simulink model "EE435_project_v10"  (R2018b)
settings: Solver=VariableStepAuto  StartTime=0.0  StopTime=8/60  RelTol=1e-3
libraries: powerlib x26, simulink x4, powerlib_meascontrol x2, re_lib x1, pePowerMeasurement x1
settings Model: Creator=jmyea  LastModifiedBy=jmyea
settings SolverCC: ZeroCrossAlgorithm=Adaptive
settings DebuggingCC: MaskedZcDiagnostic=none  IgnoredZcDiagnostic=none

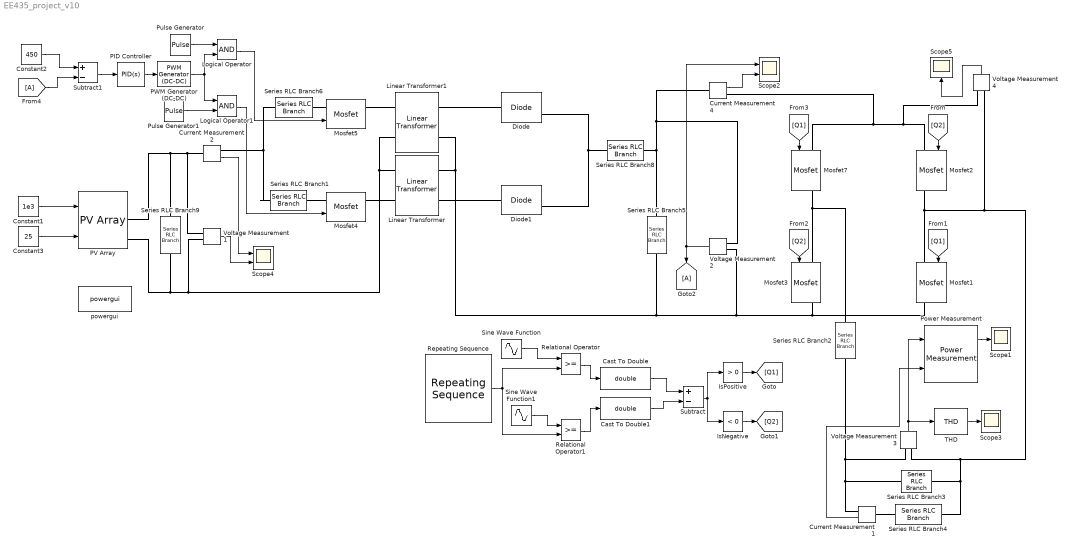
== system EE435_project_v10 ==
  Cast To Double : DataTypeConversion  OutDataTypeStr=double
  Cast To Double1 : DataTypeConversion  OutDataTypeStr=double
  Constant1 : Constant  Value=1e3
  Constant2 : Constant  Value=450
  Constant3 : Constant  Value=25
  Current Measurement1 : powerlib/Measurements/Current Measurement  PhasorSimulation=off  OutputType=Complex  PSBequivalent=0
  Current Measurement2 : powerlib/Measurements/Current Measurement  PhasorSimulation=off  OutputType=Complex  PSBequivalent=0
  Current Measurement4 : powerlib/Measurements/Current Measurement  PhasorSimulation=off  OutputType=Complex  PSBequivalent=0
  Diode : powerlib/Power Electronics/Diode  Ron=0.001  Lon=0  Vf=0.8  IC=0  UseSnubber=0  Rs=500  Cs=250e-9  Measurements=on
  Diode1 : powerlib/Power Electronics/Diode  Ron=0.001  Lon=0  Vf=0.8  IC=0  UseSnubber=0  Rs=500  Cs=250e-9  Measurements=on
  IsNegative : simulink/Logic and Bit Operations/Compare To Zero  relop=<  OutDataTypeStr=boolean
  IsPositive : simulink/Logic and Bit Operations/Compare To Zero  relop=>  OutDataTypeStr=boolean
  Linear Transformer : powerlib/Elements/Linear Transformer  UNITS=SI  NominalPower=[8.5e3 100e3]  winding1=[200 0 0]  winding2=[600 0 0]  ThreeWindings=off  winding3=[2.6e3 0 0]  RmLm=[inf inf]  Measurements=None  DataType=on
  Linear Transformer1 : powerlib/Elements/Linear Transformer  UNITS=SI  NominalPower=[8.5e3 100e3]  winding1=[200 0 0]  winding2=[600 0 0]  ThreeWindings=off  winding3=[2.6e3 0 0]  RmLm=[inf inf]  Measurements=None  DataType=on
  Logical Operator : Logic  AllPortsSameDT=off  OutDataTypeStr=boolean
  Logical Operator1 : Logic  AllPortsSameDT=off  OutDataTypeStr=boolean
  Mosfet{1..4,7} (5 alike) : powerlib/Power Electronics/Mosfet  Ron=80e-3  Lon=0  Rd=0.01  Vfd=3.5  IC=0  Rs=65.24  Cs=0.647e-6  Measurements=on
  Mosfet5 : powerlib/Power Electronics/Mosfet  Ron=80e-3  Lon=0  Rd=0.01  Vfd=3.5  IC=0  Rs=183  Cs=9.323e-9  Measurements=on
  PID Controller : simulink/Continuous/PID Controller  Controller=PID  Form=Parallel  TimeDomain=Continuous-time  SampleTime=-1  IntegratorMethod=Forward Euler  FilterMethod=Forward Euler  ControllerParametersSource=internal  P=1  I=1  D=0  UseFilter=on  N=100  TunerSelectOption=Transfer Function Based (PID Tuner App)  InitialConditionSource=internal  InitialConditionForIntegrator=0  InitialConditionForFilter=0  DifferentiatorICPrevScaledInput=0  ExternalReset=none  TrackingMode=off  Kt=1  LimitOutput=off  UpperSaturationLimit=inf  LowerSaturationLimit=-inf  LinearizeAsGain=on  AntiWindupMode=none  Kb=1  POutMin=[]  POutMax=[]  IOutMin=[]  IOutMax=[]  DOutMin=[]  DOutMax=[]  NOutMin=[]  NOutMax=[]  SumOutMin=[]  SumOutMax=[]  SaturationOutMin=[]  SaturationOutMax=[]  PParamMin=[]  PParamMax=[]  IParamMin=[]  IParamMax=[]  DParamMin=[]  DParamMax=[]  NParamMin=[]  NParamMax=[]  KbParamMin=[]  KbParamMax=[]  KtParamMin=[]  KtParamMax=[]  KbOutMin=[]  KbOutMax=[]  KtOutMin=[]  KtOutMax=[]  IntegratorOutMin=[]  IntegratorOutMax=[]  FilterOutMin=[]  FilterOutMax=[]  SumI1OutMin=[]  SumI1OutMax=[]  SumI2OutMin=[]  SumI2OutMax=[]  SumI3OutMin=[]  SumI3OutMax=[]  SumI4OutMin=[]  SumI4OutMax=[]  SumDOutMin=[]  SumDOutMax=[]  DifferentiatorOutMin=[]  DifferentiatorOutMax=[]  FilterDiffOutCoefMin=[]  FilterDiffOutCoefMax=[]  ReciprocalOutMin=[]  ReciprocalOutMax=[]  SumDenOutMin=[]  SumDenOutMax=[]  SumNumOutMin=[]  SumNumOutMax=[]  DivideOutMin=[]  DivideOutMax=[]  IntegratorContinuousStateAttributes=''  IntegratorStateMustResolveToSignalObject=off  IntegratorRTWStateStorageClass=Auto  FilterContinuousStateAttributes=''  FilterStateMustResolveToSignalObject=off  FilterRTWStateStorageClass=Auto  ParallelPVariant=InternalParameters  IdealPVariant=Disabled  IVariant=InternalParameters  DVariant=InternalParameters  IntegratorVariant=Continuous  SatVariant=Disabled  AWVariant=Passthrough  PCopyVariant=Disabled  TRVariant=Disabled  FdbkBlocksVariant=Forward  IdealPFdbkVariant=Disabled  SatFdbkVariant=Disabled  DerivativeFilterVariant=ContFilter  NVariant=InternalParameters  NCopyVariant=Disabled  FilterICVariant=InternalICsFilter  IntegratorICVariant=InternalICs  ExternalResetVariant=Disabled  TRSumVariant=Passthrough  SumFdbkVariant=Disabled  SumVariant=Sum_PID
  PV Array : re_lib/Solar/PV Array  Npar=2  Nser=5  PlotType=array @ 25 deg.C & specified irradiances  S_vec="[ 1000  500  100 ]"  Temp_C_vec="[ 45 25  ]"  ModuleName=User-defined  PlotWhenSelected=off  Pm=330.6  Ncell=60  Voc=67.7  Isc=6.07  Vm=58  Im=5.7  beta_Voc_pc=-0.276  alpha_Isc_pc=0.059  beta_Voc=-0.18685  alpha_Isc=0.0035813  IL=6.1233  I0=7.4689e-12  nI=1.6029  Rsh=328.5492  Rs=0.31806  BAL=on  Tc=1e-6  Tfilter=5e-5
  PWM Generator (DC-DC) : powerlib_meascontrol/Pulse & Signal Generators/PWM Generator (DC-DC)  Fsw=60e3  Ts=0
  Power Measurement : pePowerMeasurement/Power Measurement  LabelModeActiveChoice=Continuous  F=60  K=[0 1 2 3]  Ts=0
  Pulse Generator : DiscretePulseGenerator  PulseType=Time based  Period=1/30e3  PulseWidth=50
  Pulse Generator1 : DiscretePulseGenerator  PulseType=Time based  Period=1/30e3  PulseWidth=50  PhaseDelay=1/(2*(30e3))
  Relational Operator : RelationalOperator  OutDataTypeStr=boolean  RndMeth=Simplest
  Relational Operator1 : RelationalOperator  OutDataTypeStr=boolean  RndMeth=Simplest
  Repeating Sequence : simulink/Sources/Repeating Sequence  rep_seq_t=[0 1/(60e3) 2/(60e3) 3/(60e3) 4/(60e3)]  rep_seq_y=[1 0 -1 0 1]
  Scope1 : Scope
  Scope2 : Scope  NumInputPorts=2
  Scope3 : Scope
  Scope4 : Scope  NumInputPorts=2
  Scope5 : Scope
  Series RLC Branch1 : powerlib/Elements/Series RLC Branch  LConnTagsString=__new0  RConnTagsString=__new0  BranchType=RL  Resistance=20  Inductance=1e-3  SetiL0=off  InitialCurrent=0  Capacitance=8e-6  Setx0=off  InitialVoltage=0  Measurements=None
  Series RLC Branch2 : powerlib/Elements/Series RLC Branch  LConnTagsString=__new0  RConnTagsString=__new0  BranchType=L  Resistance=3e3  Inductance=152.78e-3  SetiL0=off  InitialCurrent=0  Capacitance=8e-6  Setx0=off  InitialVoltage=0  Measurements=None
  Series RLC Branch3 : powerlib/Elements/Series RLC Branch  LConnTagsString=__new0  RConnTagsString=__new0  BranchType=C  Resistance=100  Inductance=1E-3  SetiL0=off  InitialCurrent=0  Capacitance=46.06e-6  Setx0=off  InitialVoltage=0  Measurements=None
  Series RLC Branch4 : powerlib/Elements/Series RLC Branch  LConnTagsString=__new0  RConnTagsString=__new0  BranchType=R  Resistance=100  Inductance=7e-3  SetiL0=off  InitialCurrent=0  Capacitance=1e-6  Setx0=off  InitialVoltage=0  Measurements=None
  Series RLC Branch5 : powerlib/Elements/Series RLC Branch  LConnTagsString=__new0  RConnTagsString=__new0  BranchType=C  Resistance=3e3  Inductance=1E-3  SetiL0=off  InitialCurrent=0  Capacitance=300e-6  Setx0=off  InitialVoltage=0  Measurements=None
  Series RLC Branch6 : powerlib/Elements/Series RLC Branch  LConnTagsString=__new0  RConnTagsString=__new0  BranchType=RL  Resistance=20  Inductance=1e-3  SetiL0=off  InitialCurrent=0  Capacitance=8e-6  Setx0=off  InitialVoltage=0  Measurements=None
  Series RLC Branch8 : powerlib/Elements/Series RLC Branch  LConnTagsString=__new0  RConnTagsString=__new0  BranchType=L  Resistance=3e3  Inductance=1e-3  SetiL0=off  InitialCurrent=0  Capacitance=8e-6  Setx0=off  InitialVoltage=0  Measurements=None
  Series RLC Branch9 : powerlib/Elements/Series RLC Branch  LConnTagsString=__new0  RConnTagsString=__new0  BranchType=C  Resistance=3e3  Inductance=1E-3  SetiL0=off  InitialCurrent=0  Capacitance=50e-5  Setx0=off  InitialVoltage=0  Measurements=None
  Sine Wave Function : Sin  Amplitude=0.8  Frequency=120*pi  SampleTime=0
  Sine Wave Function1 : Sin  Amplitude=0.8  Frequency=120*pi  Phase=pi  SampleTime=0
  Subtract : Sum  Inputs=+-
  Subtract1 : Sum  Inputs=+-
  THD : powerlib_meascontrol/Measurements/THD  Freq=60  Ts=0
  Voltage Measurement{1..4} (4 alike) : powerlib/Measurements/Voltage Measurement  PhasorSimulation=off  OutputType=Complex  PSBequivalent=0
  powergui : powerlib/powergui  Priority=1  SimulationMode=Continuous  SampleTime=50e-6  frequency=60  Iterations=50  frequencyindice=0  Pbase=100e6  ErrMax=1e-4  UnitsV=kV  UnitsW=MW  buscounter=0  FunctionMessages=off  echomessages=off  EnableUseOfTLC=off  CurrentSourceSwitches=off  DisableSnubberDevices=off  DisableRonSwitches=off  DisableVfSwitches=off  DisplayEquations=off  SolverType=Tustin/Backward Euler (TBE)  Interpol=off  ExternalGateDelay=off  methode=off  Ts=100  x0status=blocks  SPID=on  SwTol=0  HookPort=off  RestoreLinks=warning  ResistiveCurrentMeasurement=off  Frange=[0:2:500]  Ylog=off  Xlog=on  ShowGrid=off  save=off  variable=ZData  structure=0  ZoomFFT=off  StartTime=0.0  cycles=1  DisplayStyle=1  fundamental=60  FreqAxis=off  MaxFrequency=1000  frequencyindicesteady=1  RmsSteady=1  display=off
  wires:
  Sine Wave Function1/1 -> Relational Operator1/1
  Subtract/1 -> IsPositive/1, IsNegative/1
  Cast To Double/1 -> Subtract/1
  [Q2] -> Mosfet3/1
  [Q2] -> Mosfet2/1
  Sine Wave Function/1 -> Relational Operator/1
  Repeating Sequence/1 -> Relational Operator1/2, Relational Operator/2
  IsNegative/1 -> [Q2]
  [Q1] -> Mosfet7/1
  Relational Operator/1 -> Cast To Double/1
  [Q1] -> Mosfet1/1
  Cast To Double1/1 -> Subtract/2
  Relational Operator1/1 -> Cast To Double1/1
  Pulse Generator/1 -> Logical Operator/1
  PWM Generator (DC-DC)/1 -> Logical Operator1/1, Logical Operator/2
  PID Controller/1 -> PWM Generator (DC-DC)/1
  Constant3/1 -> PV Array/2
  Logical Operator/1 -> Mosfet5/1
  Constant2/1 -> Subtract1/1
  Constant1/1 -> PV Array/1
  [A] -> Subtract1/2
  Logical Operator1/1 -> Mosfet4/1
  Pulse Generator1/1 -> Logical Operator1/2
  Subtract1/1 -> PID Controller/1
  IsPositive/1 -> [Q1]
  Voltage Measurement3/1 -> Power Measurement/1, THD/1
  THD/1 -> Scope3/1
  Voltage Measurement2/1 -> Scope2/1, [A]
  Current Measurement4/1 -> Scope2/2
  Current Measurement1/1 -> Power Measurement/2
  Voltage Measurement4/1 -> Scope5/1
  Voltage Measurement1/1 -> Scope4/2
  Current Measurement2/1 -> Scope4/1
  Power Measurement/1 -> Scope1/1
  connections:
  Voltage Measurement3/LConn1 -- Mosfet2/RConn1 -- Mosfet1/LConn1 -- Voltage Measurement4/LConn2 -- Series RLC Branch4/RConn1 -- Series RLC Branch3/RConn1
  Series RLC Branch8/RConn1 -- Series RLC Branch5/LConn1 -- Voltage Measurement2/LConn1 -- Current Measurement4/LConn1
  Series RLC Branch8/LConn1 -- Diode1/RConn1 -- Diode/RConn1
  Voltage Measurement1/LConn1 -- Series RLC Branch9/LConn1 -- PV Array/RConn1 -- Current Measurement2/LConn1
  Voltage Measurement2/LConn2 -- Mosfet3/RConn1 -- Mosfet1/RConn1 -- Linear Transformer1/RConn2 -- Linear Transformer/RConn1 -- Series RLC Branch5/RConn1
  PV Array/RConn2 -- Series RLC Branch9/RConn1 -- Linear Transformer1/LConn2 -- Linear Transformer/LConn1 -- Voltage Measurement1/LConn2
  Mosfet5/RConn1 -- Linear Transformer1/LConn1
  Diode/LConn1 -- Linear Transformer1/RConn1
  Mosfet4/RConn1 -- Linear Transformer/LConn2
  Series RLC Branch4/LConn1 -- Current Measurement1/LConn1
  Voltage Measurement3/LConn2 -- Series RLC Branch2/RConn1 -- Series RLC Branch3/LConn1 -- Current Measurement1/RConn1
  Mosfet3/LConn1 -- Mosfet7/RConn1 -- Series RLC Branch2/LConn1
  Diode1/LConn1 -- Linear Transformer/RConn2
  Current Measurement2/RConn1 -- Series RLC Branch1/LConn1 -- Series RLC Branch6/LConn1
  Current Measurement4/RConn1 -- Voltage Measurement4/LConn1 -- Mosfet2/LConn1 -- Mosfet7/LConn1
  Mosfet4/LConn1 -- Series RLC Branch1/RConn1
  Series RLC Branch6/RConn1 -- Mosfet5/LConn1
